simulink model "qraw2PWMmapDemo"  (R2016a)
settings: Solver=ode5  StartTime=0.0  StopTime=inf  FixedStep=0.001  RelTol=1e-3
libraries: simulink x4
settings Model: SimulationMode=external  Creator=julianleland  LastModifiedBy=julianleland
settings HardwareCC: ProdBitPerLong=64  ProdLargestAtomicFloat=None  ProdHWDeviceType=Intel->x86-64  TargetBitPerLong=64  TargetBitPerPointer=64  TargetIntDivRoundTo=Zero  TargetEndianess=LittleEndian  TargetWordSize=64  TargetHWDeviceType=Intel->x86-64
settings RTWCC: SystemTargetFile=sldrt.tlc  TemplateMakefile=sldrt.tmf  Description=Simulink Desktop Real-Time  RTWCompilerOptimization=on
settings CodeAppCC: MaxIdLength=95
settings SimulinkDesktopRealTimeCC: TargetPreCompLibLocation=/Applications/MATLAB_R2016a.app/toolbox/sldrt/lib/maci64  TargetLangStandard=C89/C90 (ANSI)  SupportVariableSizeSignals=off

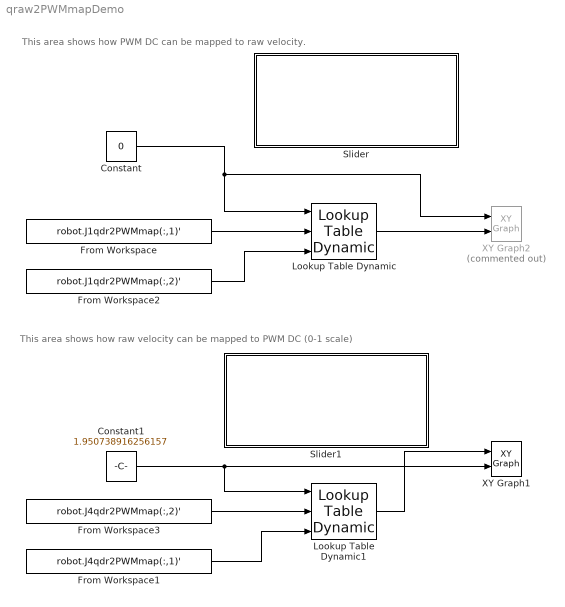
== system qraw2PWMmapDemo ==
  note: This area shows how PWM DC can be mapped to raw velocity.
  note: This area shows how raw velocity can be mapped to PWM DC (0-1 scale)
  Constant : Constant  Value=0
  Constant1 : Constant  Value=1.950738916256157
  From Workspace : FromWorkspace  VariableName=robot.J1qdr2PWMmap(:,1)'  SampleTime=0
  From Workspace1 : FromWorkspace  VariableName=robot.J4qdr2PWMmap(:,1)'  SampleTime=0
  From Workspace2 : FromWorkspace  VariableName=robot.J1qdr2PWMmap(:,2)'  SampleTime=0
  From Workspace3 : FromWorkspace  VariableName=robot.J4qdr2PWMmap(:,2)'  SampleTime=0
  Lookup Table Dynamic : simulink/Lookup Tables/Lookup Table Dynamic  LookUpMeth=Interpolation-Use End Values  OutDataTypeStr=fixdt('double')  OutputDataTypeScalingMode=Specify via dialog  OutDataType=fixdt('double')  OutScaling=2^-10  DoSatur=off
  Lookup Table Dynamic1 : simulink/Lookup Tables/Lookup Table Dynamic  LookUpMeth=Interpolation-Use End Values  OutDataTypeStr=fixdt('double')  OutputDataTypeScalingMode=Specify via dialog  OutDataType=fixdt('double')  OutScaling=2^-10  DoSatur=off
  Slider : Subsystem  DialogController=hmiCreateDDGDialog  IsWebBlock=on  mask(MWDashboardBlock){webBlockId=4649738f-3700-45d9-9de2-d2451240e4a3, webBlockType=slider, ShowInLibBrowser=on, ShowInitialText=on, HMISrcModelName=qraw2PWMmapDemo}
      mask prompts: webBlockId "WebBlock Id"; webBlockType "WebBlock Type"; HMISrcModelName "Source Model"
      mask Help: helpview([docroot '/mapfiles/simulink.map'], 'hmi_slider')
      mask Display:
      | if strcmp(get_param(bdroot(gcb),'BlockDiagramType'), 'library')
      |     image([(matlabroot) '/toolbox/simulink/hmi/icons/Slider.png']);
      | end
  Slider1 : Subsystem  DialogController=hmiCreateDDGDialog  IsWebBlock=on  mask(MWDashboardBlock){webBlockId=960520d4-fc12-4efb-adc9-d240e360649b, webBlockType=slider, ShowInLibBrowser=on, ShowInitialText=on, HMISrcModelName=qraw2PWMmapDemo}
      mask prompts: webBlockId "WebBlock Id"; webBlockType "WebBlock Type"; HMISrcModelName "Source Model"
      mask Help: helpview([docroot '/mapfiles/simulink.map'], 'hmi_slider')
      mask Display:
      | if strcmp(get_param(bdroot(gcb),'BlockDiagramType'), 'library')
      |     image([(matlabroot) '/toolbox/simulink/hmi/icons/Slider.png']);
      | end
  XY Graph1 : simulink/Sinks/XY Graph  xmin=-0.1  xmax=1.1  ymin=-2  ymax=2  st=-1
  XY Graph2 : simulink/Sinks/XY Graph  Commented=on  xmin=-0.1  xmax=1.1  ymin=-20000  ymax=20000  st=-1
  wires:
  Constant/1 -> XY Graph2/1, Lookup Table Dynamic/1
  From Workspace/1 -> Lookup Table Dynamic/2
  From Workspace2/1 -> Lookup Table Dynamic/3
  Constant1/1 -> Lookup Table Dynamic1/1, XY Graph1/2
  Lookup Table Dynamic1/1 -> XY Graph1/1
  From Workspace3/1 -> Lookup Table Dynamic1/2
  From Workspace1/1 -> Lookup Table Dynamic1/3
  Lookup Table Dynamic/1 -> XY Graph2/2

== system qraw2PWMmapDemo/Slider ==

== system qraw2PWMmapDemo/Slider1 ==
